simulink model "helicopter_control_xplane_9"  (R2016a)
settings: Solver=VariableStepAuto  StartTime=0.0  StopTime=inf  RelTol=1e-3
undefined symbols (not defined in the file): PSICMD, VyCMD
libraries: dspindex x9, dspnetwork x2, etargetslib x1
settings Model: Creator=iwin  LastModifiedBy=iwin

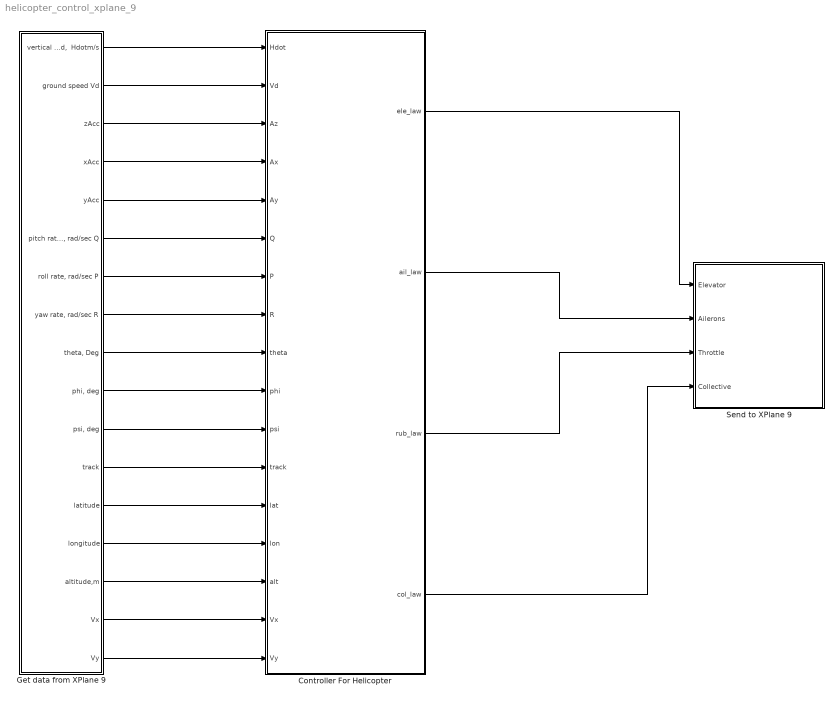
== system helicopter_control_xplane_9 ==
  Controller For Helicopter : Subsystem  mask(Controller for Helicoper){HCMD=12}
      mask prompts: HCMD "The Height CMD"
      mask help: Control the Helicopter in X-Plane 9
  Get data from XPlane 9 : Subsystem  Description=|  TreatAsAtomicUnit=on  mask(Get Data from Xplane10){remoteURL='127.0.0.1', localPort=49005, sampletime=0.02}
      | Done by: Mohamed Abdelkader
      | Contact for updates: mohamedashraf123@gmail.com
      mask prompts: remoteURL "Remote IP address ('0.0.0.0' to accept all):(default='127.0.0.1')"; localPort "Local IP port: that Xplane10 sends to (default=49005)"; sampletime "Sampling time (seconds), how frequenlty to capture data from Xplane. Don't set to low as it might not be able to capture the smaples from Xplane. Default is 0.02 assuming the UDP rate in Xplane is set to 50 sample per second"
      mask help:
      | Get Data from X-Plane10
      | * make sure you configure the right port
      | and the right IP address
      mask TypeOptions remoteURL: UDP Receive1/remoteURL
      mask TypeOptions localPort: UDP Receive1/localPort
      mask TypeOptions sampletime: UDP Receive1/sampletime
  Send to XPlane 9 : Subsystem  Description=|  mask(Send Commands to X-Plane 9){remoteURL='127.0.0.1', remotePort=49000}
      | Done by: Mohamed Abdelkader
      | Contact for updates: mohamedashraf123@gmail.com
      mask prompts: remoteURL "Remote X-Plane Address ('127.0.0.1')"; remotePort "Remote X-Plane Port (49000)"
      mask help:
      | Sends Control Surfaces Commands to Xplane 9
      | Throttle in [0,1]
      | Elevator, Ailerons, rudder, nosewheel in [-1,1]
      mask TypeOptions remoteURL: UDP Send/remoteURL
  wires:
  Controller For Helicopter/1(ele_law) -> Send to XPlane 9/1(Elevator)
  Controller For Helicopter/2(ail_law) -> Send to XPlane 9/2(Ailerons)
  Controller For Helicopter/3(rub_law) -> Send to XPlane 9/3(Throttle)
  Controller For Helicopter/4(col_law) -> Send to XPlane 9/4(Collective)
  Get data from XPlane 9/1("vertical speed,  Hdotm/s") -> Controller For Helicopter/1(Hdot)
  Get data from XPlane 9/2(ground speed Vd) -> Controller For Helicopter/2(Vd)
  Get data from XPlane 9/3(zAcc) -> Controller For Helicopter/3(Az)
  Get data from XPlane 9/4(xAcc) -> Controller For Helicopter/4(Ax)
  Get data from XPlane 9/5(yAcc) -> Controller For Helicopter/5(Ay)
  Get data from XPlane 9/6("pitch rate, rad/sec Q") -> Controller For Helicopter/6(Q)
  Get data from XPlane 9/7(" roll rate, rad/sec P") -> Controller For Helicopter/7(P)
  Get data from XPlane 9/8("yaw rate, rad/sec R") -> Controller For Helicopter/8(R)
  Get data from XPlane 9/9("theta, Deg") -> Controller For Helicopter/9(theta)
  Get data from XPlane 9/10("phi, deg") -> Controller For Helicopter/10(phi)
  Get data from XPlane 9/11("psi, deg") -> Controller For Helicopter/11(psi)
  Get data from XPlane 9/12(track) -> Controller For Helicopter/12(track)
  Get data from XPlane 9/13(latitude) -> Controller For Helicopter/13(lat)
  Get data from XPlane 9/14(longitude) -> Controller For Helicopter/14(lon)
  Get data from XPlane 9/15(altitude,m) -> Controller For Helicopter/15(alt)
  Get data from XPlane 9/16(Vx) -> Controller For Helicopter/16(Vx)
  Get data from XPlane 9/17(Vy) -> Controller For Helicopter/17(Vy)

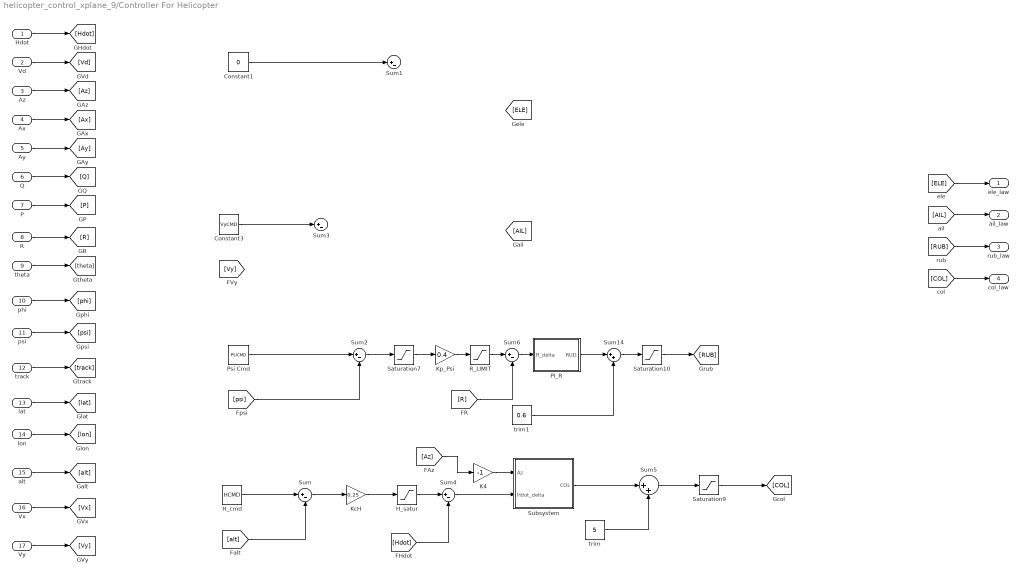
== system helicopter_control_xplane_9/Controller For Helicopter ==
  Hdot : Inport
  Vd : Inport  Port=2
  Az : Inport  Port=3
  Ax : Inport  Port=4
  Ay : Inport  Port=5
  Q : Inport  Port=6
  P : Inport  Port=7
  R : Inport  Port=8
  theta : Inport  Port=9
  phi : Inport  Port=10
  psi : Inport  Port=11
  track : Inport  Port=12
  lat : Inport  Port=13
  lon : Inport  Port=14
  alt : Inport  Port=15
  Vx : Inport  Port=16
  Vy : Inport  Port=17
  Constant1 : Constant  Value=0  OutDataTypeStr=single
  Constant3 : Constant  Value=VyCMD  OutDataTypeStr=single
  H_cmd : Constant  Value=HCMD  OutDataTypeStr=single
  H_satur : Saturate  UpperLimit=1.0  LowerLimit=-1.0
  K4 : Gain  Gain=-1
  KcH : Gain  Gain=0.25
  Kp_Psi : Gain  Gain=0.4  OutDataTypeStr=single
  PI_R : Subsystem
  Psi Cmd : Constant  Value=PSICMD  OutDataTypeStr=single
  R_LIMIT : Saturate  UpperLimit=5  LowerLimit=-5
  Saturation10 : Saturate  UpperLimit=20.0  LowerLimit=-8.0  OutDataTypeStr=single
  Saturation7 : Saturate  UpperLimit=30  LowerLimit=-30
  Saturation9 : Saturate  UpperLimit=10  LowerLimit=0
  Subsystem : Subsystem
  Sum{,1..3,6} (5 alike) : Sum  Inputs=|+-  OutDataTypeStr=double  InputSameDT=on
  Sum14 : Sum  Inputs=|++  OutMin=[-1]  OutMax=[1]  OutDataTypeStr=double  InputSameDT=on
  Sum4 : Sum  Inputs=|+-  OutDataTypeStr=single  InputSameDT=on
  Sum5 : Sum  Inputs=|++
  trim : Constant  Value=5  OutDataTypeStr=single
  trim1 : Constant  Value=0.6  OutDataTypeStr=single
  ele_law : Outport
  ail_law : Outport  Port=2
  rub_law : Outport  Port=3
  col_law : Outport  Port=4
  wires:
  H_cmd/1 -> Sum/1
  Constant1/1 -> Sum1/1
  Constant3/1 -> Sum3/1
  Psi Cmd/1 -> Sum2/1
  Hdot/1 -> [Hdot]
  Vd/1 -> [Vd]
  Az/1 -> [Az]
  Ax/1 -> [Ax]
  Ay/1 -> [Ay]
  Q/1 -> [Q]
  P/1 -> [P]
  R/1 -> [R]
  theta/1 -> [theta]
  phi/1 -> [phi]
  psi/1 -> [psi]
  track/1 -> [track]
  lat/1 -> [lat]
  lon/1 -> [lon]
  alt/1 -> [alt]
  [ELE] -> ele_law/1
  [AIL] -> ail_law/1
  [RUB] -> rub_law/1
  [COL] -> col_law/1
  [alt] -> Sum/2
  Sum/1 -> KcH/1
  Vx/1 -> [Vx]
  Vy/1 -> [Vy]
  KcH/1 -> H_satur/1
  H_satur/1 -> Sum4/1
  [Hdot] -> Sum4/2
  Sum4/1 -> Subsystem/2(Hdot_delta)
  K4/1 -> Subsystem/1(Az)
  [Az] -> K4/1
  Saturation9/1 -> [COL]
  Subsystem/1(COL) -> Sum5/1
  Sum5/1 -> Saturation9/1
  trim/1 -> Sum5/2
  [psi] -> Sum2/2
  Sum2/1 -> Saturation7/1
  Saturation7/1 -> Kp_Psi/1
  Kp_Psi/1 -> R_LIMIT/1
  R_LIMIT/1 -> Sum6/1
  [R] -> Sum6/2
  Sum6/1 -> PI_R/1(R_delta)
  PI_R/1(RUD) -> Sum14/1
  Saturation10/1 -> [RUB]
  Sum14/1 -> Saturation10/1
  trim1/1 -> Sum14/2

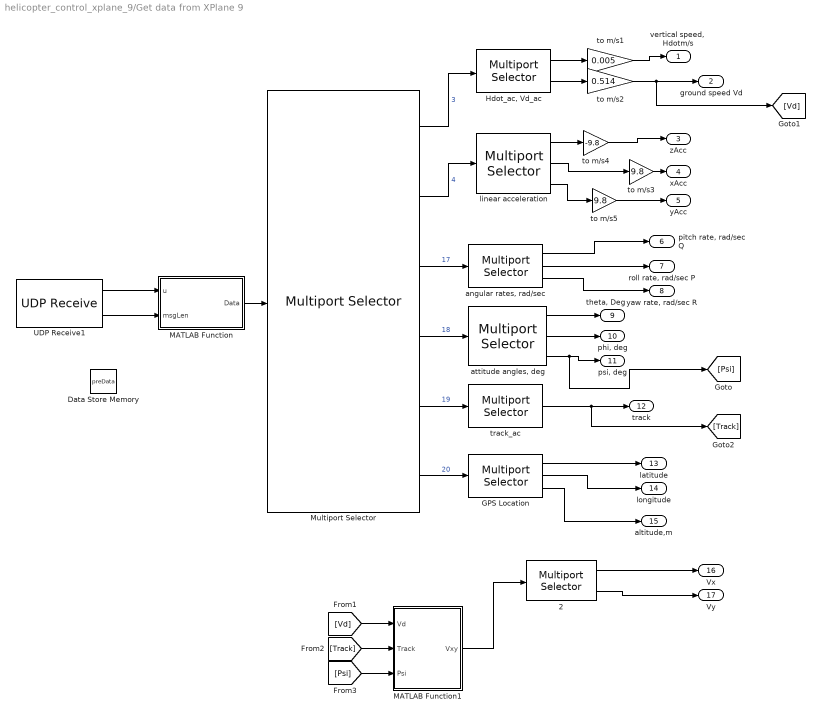
== system helicopter_control_xplane_9/Get data from XPlane 9 ==
  2 : dspindex/Multiport Selector  rowsOrCols=Columns  idxCellArray={1 2}  idxErrMode=Clip Index
  Data Store Memory : DataStoreMemory  DataStoreName=preData  InitialValue=zeros(140, 8)  ShowAdditionalParam=off  OutDataTypeStr=single
  GPS Location : dspindex/Multiport Selector  rowsOrCols=Columns  idxCellArray={1,2,3}  idxErrMode=Clip Index
  "Hdot_ac, Vd_ac" : dspindex/Multiport Selector  rowsOrCols=Columns  idxCellArray={5, 7}  idxErrMode=Clip Index
  MATLAB Function : MATLAB Function  TreatAsAtomicUnit=on
  MATLAB Function1 : MATLAB Function  TreatAsAtomicUnit=on
  Multiport Selector : dspindex/Multiport Selector  rowsOrCols=Rows  idxCellArray={3,4,17,18,20,21}  idxErrMode=Clip Index
  UDP Receive1 : dspnetwork/UDP Receive  localURL='0.0.0.0'  localPort=localPort  remoteURL=remoteURL  remotePort=-1  recvBufferSize=8192  dims=365*20  signalDatatype=uint8  isVarSize=off  showBlockingTime=off  blockingTime=0  sampletime=sampletime
  "angular rates, rad/sec" : dspindex/Multiport Selector  rowsOrCols=Columns  idxCellArray={1,2,3}  idxErrMode=Clip Index
  "attitude angles, deg" : dspindex/Multiport Selector  rowsOrCols=Columns  idxCellArray={1, 2, 3}  idxErrMode=Clip Index
  linear acceleration : dspindex/Multiport Selector  rowsOrCols=Columns  idxCellArray={3, 4, 5}  idxErrMode=Clip Index
  to m/s1 : Gain  Gain=0.005  OutDataTypeStr=double
  to m/s2 : Gain  Gain=0.514
  to m/s3 : Gain  Gain=9.8
  to m/s4 : Gain  Gain=-9.8
  to m/s5 : Gain  Gain=9.8
  track_ac : dspindex/Multiport Selector  rowsOrCols=Columns  idxCellArray={3}  idxErrMode=Clip Index
  "vertical speed,  Hdotm/s" : Outport  OutDataTypeStr=double
  ground speed Vd : Outport  Port=2
  zAcc : Outport  Port=3
  xAcc : Outport  Port=4
  yAcc : Outport  Port=5
  "pitch rate, rad/sec Q" : Outport  Port=6
  " roll rate, rad/sec P" : Outport  Port=7
  "yaw rate, rad/sec R" : Outport  Port=8
  "theta, Deg" : Outport  Port=9
  "phi, deg" : Outport  Port=10
  "psi, deg" : Outport  Port=11
  track : Outport  Port=12
  latitude : Outport  Port=13
  longitude : Outport  Port=14
  altitude,m : Outport  Port=15
  Vx : Outport  Port=16
  Vy : Outport  Port=17
  wires:
  Multiport Selector/2 -> linear acceleration/1  "4"
  "angular rates, rad/sec"/3 -> "yaw rate, rad/sec R"/1
  MATLAB Function/1(Data) -> Multiport Selector/1
  Multiport Selector/1 -> "Hdot_ac, Vd_ac"/1  "3"
  GPS Location/2 -> longitude/1
  linear acceleration/1 -> to m/s4/1
  GPS Location/1 -> latitude/1
  "angular rates, rad/sec"/2 -> " roll rate, rad/sec P"/1
  to m/s3/1 -> xAcc/1
  GPS Location/3 -> altitude,m/1
  UDP Receive1/1 -> MATLAB Function/1(u)
  UDP Receive1/2 -> MATLAB Function/2(msgLen)
  "attitude angles, deg"/3 -> [Psi], "psi, deg"/1
  "attitude angles, deg"/2 -> "phi, deg"/1
  Multiport Selector/3 -> "angular rates, rad/sec"/1  "17"
  Multiport Selector/4 -> "attitude angles, deg"/1  "18"
  Multiport Selector/5 -> track_ac/1  "19"
  Multiport Selector/6 -> GPS Location/1  "20"
  "Hdot_ac, Vd_ac"/1 -> to m/s1/1
  "Hdot_ac, Vd_ac"/2 -> to m/s2/1
  to m/s1/1 -> "vertical speed,  Hdotm/s"/1
  to m/s2/1 -> [Vd], ground speed Vd/1
  to m/s4/1 -> zAcc/1
  linear acceleration/2 -> to m/s3/1
  linear acceleration/3 -> to m/s5/1
  to m/s5/1 -> yAcc/1
  "angular rates, rad/sec"/1 -> "pitch rate, rad/sec Q"/1
  "attitude angles, deg"/1 -> "theta, Deg"/1
  track_ac/1 -> [Track], track/1
  [Psi] -> MATLAB Function1/3(Psi)
  [Track] -> MATLAB Function1/2(Track)
  [Vd] -> MATLAB Function1/1(Vd)
  MATLAB Function1/1(Vxy) -> 2/1
  2/1 -> Vx/1
  2/2 -> Vy/1

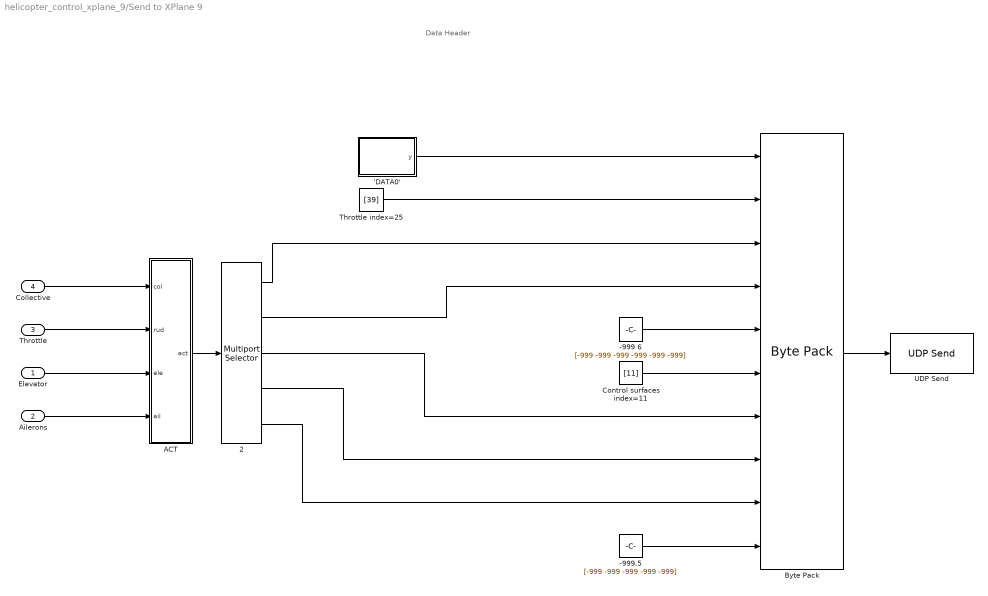
== system helicopter_control_xplane_9/Send to XPlane 9 ==
  note: Data Header
  Elevator : Inport
  Ailerons : Inport  Port=2
  Throttle : Inport  Port=3
  Collective : Inport  Port=4
  'DATA0' : MATLAB Function  TreatAsAtomicUnit=on
  -999 6 : Constant  Value=[-999 -999 -999 -999 -999 -999]  OutDataTypeStr=int32  SampleTime=-1
  -999.5 : Constant  Value=[-999 -999 -999 -999 -999]  OutDataTypeStr=int32  SampleTime=-1
  2 : dspindex/Multiport Selector  rowsOrCols=Columns  idxCellArray={1 2 3 4 5}  idxErrMode=Clip Index
  ACT : MATLAB Function  TreatAsAtomicUnit=on
  Byte Pack : etargetslib/Byte Pack  datatypes={'uint8','uint32','single','single','int32','uint32','single','single','single','int32'}  byteAlign=1
  Control surfaces index=11 : Constant  Value=[11]  OutDataTypeStr=uint32  SampleTime=-1
  Throttle index=25 : Constant  Value=[39]  OutDataTypeStr=uint32  SampleTime=-1
  UDP Send : dspnetwork/UDP Send  remoteURL=remoteURL  remotePort=49000  localURL='0.0.0.0'  localPortSource=Automatically determine  localPort=-1  sampletime=-1  separateLengthPort=0
  wires:
  Byte Pack/1 -> UDP Send/1
  Throttle index=25/1 -> Byte Pack/2
  'DATA0'/1(y) -> Byte Pack/1
  -999 6/1 -> Byte Pack/5
  Control surfaces index=11/1 -> Byte Pack/6
  -999.5/1 -> Byte Pack/10
  2/1 -> Byte Pack/3
  2/2 -> Byte Pack/4
  ACT/1(act) -> 2/1
  Collective/1 -> ACT/1(col)
  Elevator/1 -> ACT/3(ele)
  Throttle/1 -> ACT/2(rud)
  Ailerons/1 -> ACT/4(ail)
  2/3 -> Byte Pack/7
  2/4 -> Byte Pack/8
  2/5 -> Byte Pack/9

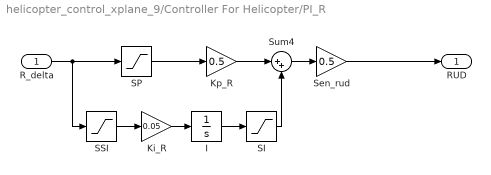
== system helicopter_control_xplane_9/Controller For Helicopter/PI_R ==
  R_delta : Inport
  I : Integrator
  Ki_R : Gain  Gain=0.05
  Kp_R : Gain  Gain=0.5
  SI : Saturate  UpperLimit=10.0  LowerLimit=-8.0
  SP : Saturate  UpperLimit=30  LowerLimit=-30
  SSI : Saturate  UpperLimit=10  LowerLimit=-10
  Sen_rud : Gain  Gain=0.5  OutDataTypeStr=single
  Sum4 : Sum  Inputs=|++  OutMin=[-20]  OutMax=[20]  OutDataTypeStr=double  InputSameDT=on
  RUD : Outport  OutDataTypeStr=single
  wires:
  SI/1 -> Sum4/2
  Kp_R/1 -> Sum4/1
  SSI/1 -> Ki_R/1
  SP/1 -> Kp_R/1
  R_delta/1 -> SSI/1, SP/1
  I/1 -> SI/1
  Ki_R/1 -> I/1
  Sum4/1 -> Sen_rud/1
  Sen_rud/1 -> RUD/1

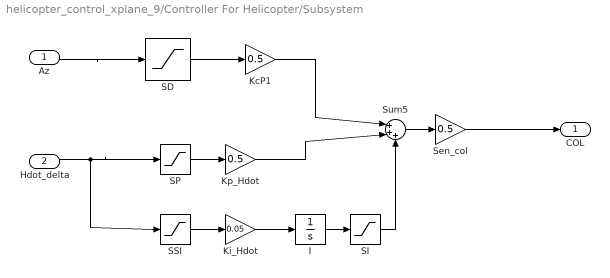
== system helicopter_control_xplane_9/Controller For Helicopter/Subsystem ==
  Az : Inport
  Hdot_delta : Inport  Port=2
  I : Integrator
  KcP1 : Gain  Gain=0.5  OutDataTypeStr=single
  Ki_Hdot : Gain  Gain=0.05  OutDataTypeStr=double
  Kp_Hdot : Gain  Gain=0.5  OutDataTypeStr=single
  SD : Saturate  UpperLimit=3.0  LowerLimit=-3.0
  SI : Saturate  UpperLimit=2.0  LowerLimit=-2.0  OutDataTypeStr=single
  SP : Saturate  UpperLimit=4.0  LowerLimit=-4.0
  SSI : Saturate  UpperLimit=1.0  LowerLimit=-1.0
  Sen_col : Gain  Gain=0.5  OutDataTypeStr=single
  Sum5 : Sum  Inputs=|+++  AccumDataTypeStr=single  OutMin=[-20]  OutMax=[20]  OutDataTypeStr=single  InputSameDT=on
  COL : Outport  OutDataTypeStr=single
  wires:
  Az/1 -> SD/1
  SD/1 -> KcP1/1
  KcP1/1 -> Sum5/1
  Hdot_delta/1 -> SSI/1, SP/1
  SSI/1 -> Ki_Hdot/1
  Ki_Hdot/1 -> I/1
  SP/1 -> Kp_Hdot/1
  Kp_Hdot/1 -> Sum5/2
  I/1 -> SI/1
  SI/1 -> Sum5/3
  Sen_col/1 -> COL/1
  Sum5/1 -> Sen_col/1

== matlab function helicopter_control_xplane_9/Get data from XPlane 9/MATLAB Function ==
  data: u input uint8; Data output single size=[140 8]; msgLen input; preData data_store_memory
% 
% Handle the data received from x-plane 9
% 
% Author: Gui Zhou
% Date: 2017-02-14
%

function Data  = fcn(u,msgLen)
    %#codegen
    global preData; 
    %coder.extrinsic('clear')
    dataLen=msgLen-5;
    Npackets=dataLen/36; 
    % initialize data matrix
    % rows: packets of data; columns: data values, first column is the data
    % index  



    maxNPackets=140;
    Nvalues=8;% number of values in each packet
    Data=single(zeros(maxNPackets,Nvalues));

    if dataLen ~= 0 

        Bytecounter=6; % start after the 5th byte 
        for j=1:Npackets
                        indx=typecast(u(Bytecounter:Bytecounter+3),'uint32');% packet index
                        %Data(indx,1)=single(indx); % packet index
                        Bytecounter=Bytecounter+4; % go to the next 4 bytes
                        Data(indx,1)=typecast(u(Bytecounter:Bytecounter+3),'single'); % 1st value
                        Bytecounter=Bytecounter+4; % go to the next 4 bytes
                        Data(indx,2)=typecast(u(Bytecounter:Bytecounter+3),'single'); % 2nd value
                        Bytecounter=Bytecounter+4; % go to the next 4 bytes
                        Data(indx,3)=typecast(u(Bytecounter:Bytecounter+3),'single'); % 3rd value
                        Bytecounter=Bytecounter+4; % go to the next 4 bytes
                        Data(indx,4)=typecast(u(Bytecounter:Bytecounter+3),'single'); % 4th value
                        Bytecounter=Bytecounter+4; % go to the next 4 bytes
                        Data(indx,5)=typecast(u(Bytecounter:Bytecounter+3),'single'); % 5th value
                        Bytecounter=Bytecounter+4; % go to the next 4 bytes
                        Data(indx,6)=typecast(u(Bytecounter:Bytecounter+3),'single'); % 6th value
                        Bytecounter=Bytecounter+4; % go to the next 4 bytes
                        Data(indx,7)=typecast(u(Bytecounter:Bytecounter+3),'single'); % 7th value
                        Bytecounter=Bytecounter+4; % go to the next 4 bytes
                        Data(indx,8)=typecast(u(Bytecounter:Bytecounter+3),'single'); % 8th value
                        Bytecounter=Bytecounter+4;% go to the next packet index 
        end  
        
        preData = Data;

    else 

        Data = preData;
   
    end
end



%clear Data

== matlab function helicopter_control_xplane_9/Send to XPlane 9/'DATA0' ==
  data: y output
function y = fcn()
%#codegen
%y=uint8(zeros(1,77));
y = uint8('DATA0');

== matlab function helicopter_control_xplane_9/Get data from XPlane 9/MATLAB Function1 ==
  data: Vd input; Vxy output size=[1 2]; Track input; Psi input
function Vxy  = fcn(Vd,Track,Psi)
    Vxy=single(zeros(1,2));
	Vxy(1,1)=Vd*cos((Track-Psi)/57.3);
	Vxy(1,2)=Vd*sin((Track-Psi)/57.3);
end
%clear Data

== matlab function helicopter_control_xplane_9/Send to XPlane 9/ACT ==
  data: act output size=[1 5]; col input; rud input; ele input; ail input
function act  = fcn(col,rud,ele,ail)
    act=single(zeros(1,5));
	act(1,1)=col;
    act(1,2)=-(rud-5.0)*2.0;
	act(1,3)=(rud-5.0)/10.0;
    act(1,4)=-(ele/5.0);
    act(1,5)=ail/5.0;
end
